simulink model "pid_control"  (R2022a)
settings: Solver=VariableStepAuto  StartTime=0.0  StopTime=10.0  RelTol=1e-3
settings Model: Creator=Administrator  LastModifiedBy=Administrator

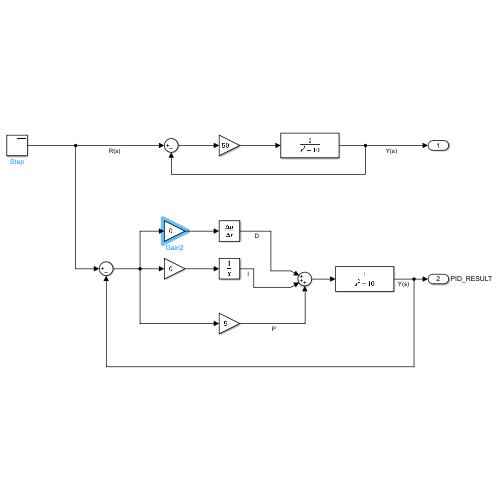
[thumbnail: Simulink's stored preview of the top-level diagram]
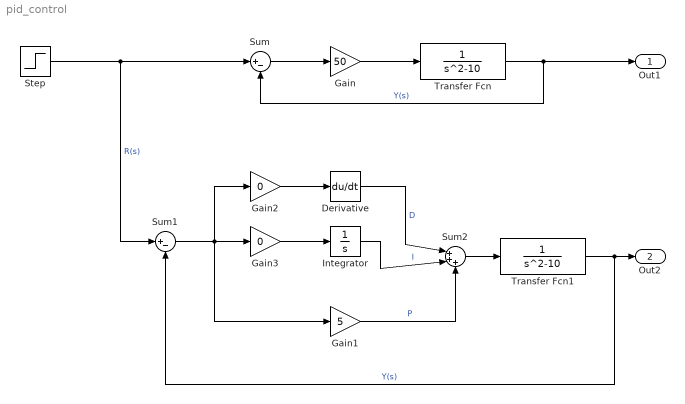
== system pid_control ==
  Derivative : Derivative
  Gain : Gain  Gain=50
  Gain1 : Gain  Gain=5
  Gain2 : Gain  Gain=0
  Gain3 : Gain  Gain=0
  Integrator : Integrator
  Step : Step  After=10  SampleTime=0
  Sum : Sum  Inputs=|+-
  Sum1 : Sum  Inputs=|+-
  Sum2 : Sum  Inputs=|+++
  Transfer Fcn : TransferFcn  Denominator=[1 0 -10]
  Transfer Fcn1 : TransferFcn  Denominator=[1 0 -10]
  Out1 : Outport
  Out2 : Outport  Port=2  SignalName=PID_RESULT
  wires:
  Step/1 -> Sum1/1, Sum/1  "R(s)"
  Sum/1 -> Gain/1
  Gain/1 -> Transfer Fcn/1
  Transfer Fcn/1 -> Sum/2, Out1/1  "Y(s)"
  Gain2/1 -> Derivative/1
  Sum2/1 -> Transfer Fcn1/1
  Derivative/1 -> Sum2/1  "D"
  Integrator/1 -> Sum2/2  "I"
  Gain1/1 -> Sum2/3  "P"
  Gain3/1 -> Integrator/1
  Sum1/1 -> Gain1/1, Gain2/1, Gain3/1
  Transfer Fcn1/1 -> Sum1/2, Out2/1  "Y(s)"
